simulink model "recycle1"  (R2024a)
settings: Solver=VariableStepAuto  StartTime=0.0  StopTime=100  MaxStep=0.1  RelTol=1e-3
libraries: simulink x20
(part 1 of 2)
settings Model: Creator=SEPTPFNK  LastModifiedBy=skoge
settings DataIOCC: SaveFormat=Array  SaveOutput=off  DSMLogging=off  ReturnWorkspaceOutputs=off  TimeSaveName=t
settings OptimizationCC: ReuseModelBlockBuffer=off
settings RTWCC: GPUComputeCapability=3.5

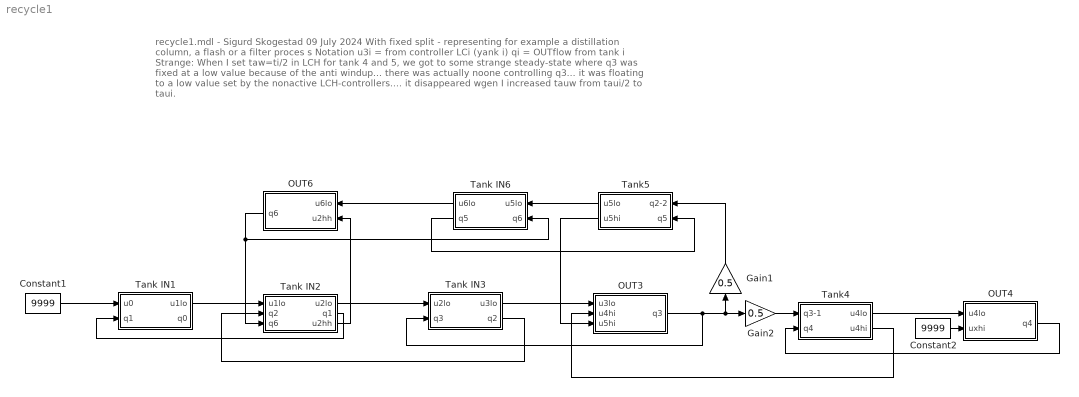
== system recycle1 ==
  note: recycle1.mdl - Sigurd Skogestad 09 July 2024
      | With fixed split - representing for example a distillation column, a flash or a filter proces s
      | Notation
      | u3i = from controller LCi (yank i)
      | qi = OUTflow from tank i
      |
      | Strange: When I set taw=ti/2 in LCH for tank 4 and 5, we got to some strange steady-state where q3 was fixed at a low value because of the anti windup... there was actually noone controlling q3... it was floating to a low value set by the nonactive LCH-controllers.... it disappeared wgen I increased tauw from taui/2 to taui.
  Constant1 : Constant  Value=9999
  Constant2 : Constant  Value=9999
  Gain1 : Gain  Gain=0.5  SaturateOnIntegerOverflow=on  OutDataTypeStr=Inherit: Same as input  ParamDataTypeStr=Inherit: Same as input
  Gain2 : Gain  Gain=0.5  SaturateOnIntegerOverflow=on  OutDataTypeStr=Inherit: Same as input  ParamDataTypeStr=Inherit: Same as input
  OUT3 : Subsystem
  OUT4 : Subsystem
  OUT6 : Subsystem
  Tank IN1 : Subsystem
  Tank IN2 : Subsystem
  Tank IN3 : Subsystem
  Tank IN6 : Subsystem
  Tank4 : Subsystem
  Tank5 : Subsystem
  wires:
  Tank IN1/1(u1lo) -> Tank IN2/1(u1lo)
  Tank IN2/2(q1) -> Tank IN1/2(q1)
  Constant1/1 -> Tank IN1/1(u0)
  Tank IN2/1(u2lo) -> Tank IN3/1(u2lo)
  Tank IN3/2(q2) -> Tank IN2/2(q2)
  Tank IN3/1(u3lo) -> OUT3/1(u3lo)
  OUT3/1(q3) -> Gain1/1, Gain2/1, Tank IN3/2(q3)
  Gain2/1 -> Tank4/1(q3-1)
  Tank4/1(u4lo) -> OUT4/1(u4lo)
  OUT4/1(q4) -> Tank4/2(q4)
  Constant2/1 -> OUT4/2(uxhi)
  Tank4/2(u4hi) -> OUT3/2(u4hi)
  Gain1/1 -> Tank5/1(q2-2)
  Tank5/2(u5hi) -> OUT3/3(u5hi)
  Tank5/1(u5lo) -> Tank IN6/1(u5lo)
  Tank IN6/2(q5) -> Tank5/2(q5)
  Tank IN6/1(u6lo) -> OUT6/1(u6lo)
  OUT6/1(q6) -> Tank IN2/3(q6), Tank IN6/2(q6)
  Tank IN2/3(u2hh) -> OUT6/2(u2hh)

== system recycle1/OUT3 ==
  note: This block represents an outflow valve and selector.
  note: Manual max-value; may represent bottleneck
  u3lo : Inport
  u4hi : Inport  Port=2
  u5hi : Inport  Port=3
  Constant2 : Constant  Value=9999
  Constant5 : Constant  Value=100
  Constant7 : Constant  Value=0
  SEL1 : MinMax  Inputs=4
  Saturation Dynamic : simulink/Discontinuities/Saturation Dynamic  OutMin=[]  OutMax=[]  OutDataTypeStr=Inherit: Same as second input  OutDataType=fixdt(1, 16)  OutScaling=2^-10  DoSatur=off
  Sum2 : Sum  Inputs=+++|
  ubq2 : Step  Time=120  After=-50  SampleTime=0
  ubq4 : Step  Time=100  After=10  SampleTime=0
  q3 : Outport
  wires:
  u3lo/1 -> SEL1/1
  SEL1/1 -> Saturation Dynamic/2
  Constant5/1 -> Saturation Dynamic/1
  Constant7/1 -> Saturation Dynamic/3
  Sum2/1 -> SEL1/2  "ubq4"
  Constant2/1 -> Sum2/1
  ubq2/1 -> Sum2/3
  ubq4/1 -> Sum2/2
  Saturation Dynamic/1 -> q3/1  "q3"
  u4hi/1 -> SEL1/3
  u5hi/1 -> SEL1/4

== system recycle1/OUT4 ==
  note: This block represents an outflow valve and selector.
  note: Manual max-value; may represent bottleneck
  u4lo : Inport
  uxhi : Inport  Port=2
  Constant2 : Constant  Value=9999
  Constant5 : Constant  Value=100
  Constant7 : Constant  Value=0
  SEL1 : MinMax  Inputs=3
  Saturation Dynamic : simulink/Discontinuities/Saturation Dynamic  OutMin=[]  OutMax=[]  OutDataTypeStr=Inherit: Same as second input  OutDataType=fixdt(1, 16)  OutScaling=2^-10  DoSatur=off
  Sum2 : Sum  Inputs=+++|
  ubq2 : Step  Time=40  After=-10  SampleTime=0
  ubq4 : Step  Time=10  After=0  SampleTime=0
  q4 : Outport
  wires:
  u4lo/1 -> SEL1/1
  SEL1/1 -> Saturation Dynamic/2
  Constant5/1 -> Saturation Dynamic/1
  Constant7/1 -> Saturation Dynamic/3
  Sum2/1 -> SEL1/2  "ubq5"
  Constant2/1 -> Sum2/1
  ubq2/1 -> Sum2/3
  ubq4/1 -> Sum2/2
  Saturation Dynamic/1 -> q4/1  "q4"
  uxhi/1 -> SEL1/3

== system recycle1/OUT6 ==
  note: This block represents an outflow valve and selector.
  note: Manual max-value; may represent bottleneck
  u6lo : Inport
  u2hh : Inport  Port=2
  Constant2 : Constant  Value=999
  Constant5 : Constant  Value=100
  Constant7 : Constant  Value=0
  SEL1 : MinMax  Inputs=3
  Saturation Dynamic : simulink/Discontinuities/Saturation Dynamic  OutMin=[]  OutMax=[]  OutDataTypeStr=Inherit: Same as second input  OutDataType=fixdt(1, 16)  OutScaling=2^-10  DoSatur=off
  Sum2 : Sum  Inputs=+++|
  ubq2 : Step  Time=40  After=-10  SampleTime=0
  ubq4 : Step  Time=10  After=0  SampleTime=0
  q6 : Outport
  wires:
  u6lo/1 -> SEL1/1
  SEL1/1 -> Saturation Dynamic/2
  Constant5/1 -> Saturation Dynamic/1
  Constant7/1 -> Saturation Dynamic/3
  Sum2/1 -> SEL1/2  "ubq5"
  Constant2/1 -> Sum2/1
  ubq2/1 -> Sum2/3
  ubq4/1 -> Sum2/2
  Saturation Dynamic/1 -> q6/1  "q7"
  u2hh/1 -> SEL1/3

== system recycle1/Tank IN1 ==
  note: This block represents a tank with bidirectional level control + inflow valve and selector.
  note: Manual max-value; may represent bottleneck
  u0 : Inport
  q1 : Inport  Port=2
  B2 : Integrator  InitialCondition=80  LimitOutput=on  UpperSaturationLimit=200  LowerSaturationLimit=-100
  Constant2 : Constant  Value=100
  Constant5 : Constant  Value=100
  Constant7 : Constant  Value=0
  LCH1 : Subsystem  mask(PID-controller){Kc=1, Ti=4, Tarw=4, r0=80, u0=80, yMin=0, yMax=100, uMin=0, uMax=100}
      mask prompts: Tarw "T_arw"; r0 "Setpoint:"; u0 "Initial output:"
      mask help: PID-controller
      mask Help:
      | <P> PID-controller with beta-factor, limiting, ARW etc </P>
      | 
      | Inputs: <P>
      |  <UL>
      |   1 = r (setpoint) <BR>
      |   2 = y (process value) <BR>
      |   3  = u0 (control signal offset) <BR>
      |  </UL>
      |  </P>
      | Outputs: <P>
      |  <UL>
      |    1 = u (control signal) <BR>
      |    2 = Proportional part  <BR>
      |    3 = Integral part  <BR>
      |    4 = Derivative part  <BR>
      |    5 = raw signal, without ARW  <BR>
      |  </UL>
      |  </P>
      mask Display:
      | disp(['PI' 10 10 10])
      | port_label('input',1,'y')
      | port_label('input',2,'uaw')
      | port_label('output',1,'u')
  LCL1 : Subsystem  mask(PID-controller){Kc=-1, Ti=4, Tarw=4, r0=10, u0=80, yMin=0, yMax=100, uMin=0, uMax=100}
      mask prompts: Tarw "T_arw"; r0 "Setpoint:"; u0 "Initial output:"
      mask help: PID-controller
      mask Help:
      | <P> PID-controller with beta-factor, limiting, ARW etc </P>
      | 
      | Inputs: <P>
      |  <UL>
      |   1 = r (setpoint) <BR>
      |   2 = y (process value) <BR>
      |   3  = u0 (control signal offset) <BR>
      |  </UL>
      |  </P>
      | Outputs: <P>
      |  <UL>
      |    1 = u (control signal) <BR>
      |    2 = Proportional part  <BR>
      |    3 = Integral part  <BR>
      |    4 = Derivative part  <BR>
      |    5 = raw signal, without ARW  <BR>
      |  </UL>
      |  </P>
      mask Display:
      | disp(['PI' 10 10 10])
      | port_label('input',1,'y')
      | port_label('input',2,'uaw')
      | port_label('output',1,'u')
  SEL1 : MinMax  Inputs=3
  Saturation Dynamic : simulink/Discontinuities/Saturation Dynamic  OutMin=[]  OutMax=[]  OutDataTypeStr=Inherit: Same as second input  OutDataType=fixdt(1, 16)  OutScaling=2^-10  DoSatur=off
  Sum1 : Sum  Inputs=|-+|
  Sum2 : Sum  Inputs=+++|
  ubq2 : Step  Time=120  After=-20  SampleTime=0
  ubq4 : Step  Time=40  After=-70  SampleTime=0
  u1lo : Outport
  q0 : Outport  Port=2
  wires:
  B2/1 -> LCL1/1(in_y), LCH1/1(in_y)  "x1"
  u0/1 -> SEL1/1
  SEL1/1 -> Saturation Dynamic/2
  Constant5/1 -> Saturation Dynamic/1
  LCH1/1(out_u) -> SEL1/3  "u1hi"
  Sum1/1 -> B2/1
  Constant7/1 -> Saturation Dynamic/3
  Saturation Dynamic/1 -> Sum1/2, q0/1, LCH1/2(in_yaw)  "q0"
  q1/1 -> LCL1/2(in_yaw), Sum1/1
  Sum2/1 -> SEL1/2  "ubq1"
  Constant2/1 -> Sum2/1
  ubq2/1 -> Sum2/3
  ubq4/1 -> Sum2/2
  LCL1/1(out_u) -> u1lo/1  "u1lo"

== system recycle1/Tank IN2 ==
  note: This block represents a tank with bidirectional level control + inflow valve and selector + t wo inflows (so one H and one HH setpoint)
  note: Manual max-value; may represent bottleneck
  u1lo : Inport
  q2 : Inport  Port=2
  q6 : Inport  Port=3
  B2 : Integrator  InitialCondition=80  LimitOutput=on  UpperSaturationLimit=200  LowerSaturationLimit=-100
  Constant2 : Constant  Value=9999
  Constant5 : Constant  Value=100
  Constant7 : Constant  Value=0
  LCH2 : Subsystem  mask(PID-controller){Kc=1, Ti=4, Tarw=4, r0=80, u0=80, yMin=0, yMax=100, uMin=0, uMax=100}
      mask prompts: Tarw "T_arw"; r0 "Setpoint:"; u0 "Initial output:"
      mask help: PID-controller
      mask Help:
      | <P> PID-controller with beta-factor, limiting, ARW etc </P>
      | 
      | Inputs: <P>
      |  <UL>
      |   1 = r (setpoint) <BR>
      |   2 = y (process value) <BR>
      |   3  = u0 (control signal offset) <BR>
      |  </UL>
      |  </P>
      | Outputs: <P>
      |  <UL>
      |    1 = u (control signal) <BR>
      |    2 = Proportional part  <BR>
      |    3 = Integral part  <BR>
      |    4 = Derivative part  <BR>
      |    5 = raw signal, without ARW  <BR>
      |  </UL>
      |  </P>
      mask Display:
      | disp(['PI' 10 10 10])
      | port_label('input',1,'y')
      | port_label('input',2,'uaw')
      | port_label('output',1,'u')
  LCHH2 : Subsystem  mask(PID-controller){Kc=1, Ti=4, Tarw=4, r0=90, u0=90, yMin=0, yMax=100, uMin=0, uMax=100}
      mask prompts: Tarw "T_arw"; r0 "Setpoint:"; u0 "Initial output:"
      mask help: PID-controller
      mask Help:
      | <P> PID-controller with beta-factor, limiting, ARW etc </P>
      | 
      | Inputs: <P>
      |  <UL>
      |   1 = r (setpoint) <BR>
      |   2 = y (process value) <BR>
      |   3  = u0 (control signal offset) <BR>
      |  </UL>
      |  </P>
      | Outputs: <P>
      |  <UL>
      |    1 = u (control signal) <BR>
      |    2 = Proportional part  <BR>
      |    3 = Integral part  <BR>
      |    4 = Derivative part  <BR>
      |    5 = raw signal, without ARW  <BR>
      |  </UL>
      |  </P>
      mask Display:
      | disp(['PI' 10 10 10])
      | port_label('input',1,'y')
      | port_label('input',2,'uaw')
      | port_label('output',1,'u')
  LCL2 : Subsystem  mask(PID-controller){Kc=-1, Ti=4, Tarw=4, r0=10, u0=80, yMin=0, yMax=100, uMin=0, uMax=100}
      mask prompts: Tarw "T_arw"; r0 "Setpoint:"; u0 "Initial output:"
      mask help: PID-controller
      mask Help:
      | <P> PID-controller with beta-factor, limiting, ARW etc </P>
      | 
      | Inputs: <P>
      |  <UL>
      |   1 = r (setpoint) <BR>
      |   2 = y (process value) <BR>
      |   3  = u0 (control signal offset) <BR>
      |  </UL>
      |  </P>
      | Outputs: <P>
      |  <UL>
      |    1 = u (control signal) <BR>
      |    2 = Proportional part  <BR>
      |    3 = Integral part  <BR>
      |    4 = Derivative part  <BR>
      |    5 = raw signal, without ARW  <BR>
      |  </UL>
      |  </P>
      mask Display:
      | disp(['PI' 10 10 10])
      | port_label('input',1,'y')
      | port_label('input',2,'uaw')
      | port_label('output',1,'u')
  SEL1 : MinMax  Inputs=3
  Saturation Dynamic : simulink/Discontinuities/Saturation Dynamic  OutMin=[]  OutMax=[]  OutDataTypeStr=Inherit: Same as second input  OutDataType=fixdt(1, 16)  OutScaling=2^-10  DoSatur=off
  Sum1 : Sum  Inputs=|-++|
  Sum2 : Sum  Inputs=+++|
  ubq2 : Step  Time=120  After=-20  SampleTime=0
  ubq4 : Step  Time=102  After=20  SampleTime=0
  u2lo : Outport
  q1 : Outport  Port=2
  u2hh : Outport  Port=3
  wires:
  B2/1 -> LCHH2/1(in_y), LCL2/1(in_y), LCH2/1(in_y)  "x2"
  u1lo/1 -> SEL1/1
  SEL1/1 -> Saturation Dynamic/2
  Constant5/1 -> Saturation Dynamic/1
  LCH2/1(out_u) -> SEL1/3  "u2hi"
  Sum1/1 -> B2/1
  Constant7/1 -> Saturation Dynamic/3
  Saturation Dynamic/1 -> LCH2/2(in_yaw), Sum1/2, q1/1  "q1"
  q2/1 -> LCL2/2(in_yaw), Sum1/1
  Sum2/1 -> SEL1/2  "ubq2"
  Constant2/1 -> Sum2/1
  ubq2/1 -> Sum2/3
  ubq4/1 -> Sum2/2
  LCL2/1(out_u) -> u2lo/1  "u2lo"
  LCHH2/1(out_u) -> u2hh/1  "u2hh"
  q6/1 -> LCHH2/2(in_yaw), Sum1/3

== system recycle1/Tank IN3 ==
  note: This block represents a tank with bidirectional level control + inflow valve and selector.
  note: Manual max-value; may represent bottleneck
  u2lo : Inport
  q3 : Inport  Port=2
  B3 : Integrator  InitialCondition=80  LimitOutput=on  UpperSaturationLimit=200  LowerSaturationLimit=-100
  Constant2 : Constant  Value=9999
  Constant5 : Constant  Value=100
  Constant7 : Constant  Value=0
  LCH3 : Subsystem  mask(PID-controller){Kc=1, Ti=4, Tarw=4, r0=80, u0=80, yMin=0, yMax=100, uMin=0, uMax=100}
      mask prompts: Tarw "T_arw"; r0 "Setpoint:"; u0 "Initial output:"
      mask help: PID-controller
      mask Help:
      | <P> PID-controller with beta-factor, limiting, ARW etc </P>
      | 
      | Inputs: <P>
      |  <UL>
      |   1 = r (setpoint) <BR>
      |   2 = y (process value) <BR>
      |   3  = u0 (control signal offset) <BR>
      |  </UL>
      |  </P>
      | Outputs: <P>
      |  <UL>
      |    1 = u (control signal) <BR>
      |    2 = Proportional part  <BR>
      |    3 = Integral part  <BR>
      |    4 = Derivative part  <BR>
      |    5 = raw signal, without ARW  <BR>
      |  </UL>
      |  </P>
      mask Display:
      | disp(['PI' 10 10 10])
      | port_label('input',1,'y')
      | port_label('input',2,'uaw')
      | port_label('output',1,'u')
  LCL3 : Subsystem  mask(PID-controller){Kc=-1, Ti=4, Tarw=4, r0=10, u0=80, yMin=0, yMax=100, uMin=0, uMax=100}
      mask prompts: Tarw "T_arw"; r0 "Setpoint:"; u0 "Initial output:"
      mask help: PID-controller
      mask Help:
      | <P> PID-controller with beta-factor, limiting, ARW etc </P>
      | 
      | Inputs: <P>
      |  <UL>
      |   1 = r (setpoint) <BR>
      |   2 = y (process value) <BR>
      |   3  = u0 (control signal offset) <BR>
      |  </UL>
      |  </P>
      | Outputs: <P>
      |  <UL>
      |    1 = u (control signal) <BR>
      |    2 = Proportional part  <BR>
      |    3 = Integral part  <BR>
      |    4 = Derivative part  <BR>
      |    5 = raw signal, without ARW  <BR>
      |  </UL>
      |  </P>
      mask Display:
      | disp(['PI' 10 10 10])
      | port_label('input',1,'y')
      | port_label('input',2,'uaw')
      | port_label('output',1,'u')
  SEL1 : MinMax  Inputs=3
  Saturation Dynamic : simulink/Discontinuities/Saturation Dynamic  OutMin=[]  OutMax=[]  OutDataTypeStr=Inherit: Same as second input  OutDataType=fixdt(1, 16)  OutScaling=2^-10  DoSatur=off
  Sum1 : Sum  Inputs=|-+|
  Sum2 : Sum  Inputs=+++|
  ubq2 : Step  Time=20  After=-60  SampleTime=0
  ubq4 : Step  Time=10  After=20  SampleTime=0
  u3lo : Outport
  q2 : Outport  Port=2
  wires:
  B3/1 -> LCH3/1(in_y), LCL3/1(in_y)  "x3"
  u2lo/1 -> SEL1/1
  SEL1/1 -> Saturation Dynamic/2
  Constant5/1 -> Saturation Dynamic/1
  LCH3/1(out_u) -> SEL1/3  "u3hi"
  Sum1/1 -> B3/1
  Constant7/1 -> Saturation Dynamic/3
  Saturation Dynamic/1 -> LCH3/2(in_yaw), Sum1/2, q2/1  "q2"
  q3/1 -> LCL3/2(in_yaw), Sum1/1
  Sum2/1 -> SEL1/2  "ubq3"
  Constant2/1 -> Sum2/1
  ubq2/1 -> Sum2/3
  ubq4/1 -> Sum2/2
  LCL3/1(out_u) -> u3lo/1  "u3lo"

== system recycle1/Tank IN6 ==
  note: This block represents a tank with bidirectional level control + inflow valve and selector.
  note: Manual max-value; may represent bottleneck
  u5lo : Inport
  q6 : Inport  Port=2
  B6 : Integrator  InitialCondition=10  LimitOutput=on  UpperSaturationLimit=200  LowerSaturationLimit=-100
  Constant2 : Constant  Value=100
  Constant5 : Constant  Value=100
  Constant7 : Constant  Value=0
  LCH6 : Subsystem  mask(PID-controller){Kc=1, Ti=4, Tarw=4, r0=80, u0=80, yMin=0, yMax=100, uMin=0, uMax=100}
      mask prompts: Tarw "T_arw"; r0 "Setpoint:"; u0 "Initial output:"
      mask help: PID-controller
      mask Help:
      | <P> PID-controller with beta-factor, limiting, ARW etc </P>
      | 
      | Inputs: <P>
      |  <UL>
      |   1 = r (setpoint) <BR>
      |   2 = y (process value) <BR>
      |   3  = u0 (control signal offset) <BR>
      |  </UL>
      |  </P>
      | Outputs: <P>
      |  <UL>
      |    1 = u (control signal) <BR>
      |    2 = Proportional part  <BR>
      |    3 = Integral part  <BR>
      |    4 = Derivative part  <BR>
      |    5 = raw signal, without ARW  <BR>
      |  </UL>
      |  </P>
      mask Display:
      | disp(['PI' 10 10 10])
      | port_label('input',1,'y')
      | port_label('input',2,'uaw')
      | port_label('output',1,'u')
  LCL6 : Subsystem  mask(PID-controller){Kc=-1, Ti=4, Tarw=4, r0=10, u0=80, yMin=0, yMax=100, uMin=0, uMax=100}
      mask prompts: Tarw "T_arw"; r0 "Setpoint:"; u0 "Initial output:"
      mask help: PID-controller
      mask Help:
      | <P> PID-controller with beta-factor, limiting, ARW etc </P>
      | 
      | Inputs: <P>
      |  <UL>
      |   1 = r (setpoint) <BR>
      |   2 = y (process value) <BR>
      |   3  = u0 (control signal offset) <BR>
      |  </UL>
      |  </P>
      | Outputs: <P>
      |  <UL>
      |    1 = u (control signal) <BR>
      |    2 = Proportional part  <BR>
      |    3 = Integral part  <BR>
      |    4 = Derivative part  <BR>
      |    5 = raw signal, without ARW  <BR>
      |  </UL>
      |  </P>
      mask Display:
      | disp(['PI' 10 10 10])
      | port_label('input',1,'y')
      | port_label('input',2,'uaw')
      | port_label('output',1,'u')
  SEL1 : MinMax  Inputs=3
  Saturation Dynamic : simulink/Discontinuities/Saturation Dynamic  OutMin=[]  OutMax=[]  OutDataTypeStr=Inherit: Same as second input  OutDataType=fixdt(1, 16)  OutScaling=2^-10  DoSatur=off
  Sum1 : Sum  Inputs=|-+|
  Sum2 : Sum  Inputs=+++|
  ubq2 : Step  Time=200  After=-60  SampleTime=0
  ubq4 : Step  Time=60  After=-90  SampleTime=0
  u6lo : Outport
  q5 : Outport  Port=2
  wires:
  B6/1 -> LCH6/1(in_y), LCL6/1(in_y)  "x6"
  u5lo/1 -> SEL1/1
  SEL1/1 -> Saturation Dynamic/2
  Constant5/1 -> Saturation Dynamic/1
  LCH6/1(out_u) -> SEL1/3  "u6hi"
  Sum1/1 -> B6/1
  Constant7/1 -> Saturation Dynamic/3
  Saturation Dynamic/1 -> LCH6/2(in_yaw), Sum1/2, q5/1  "q5"
  q6/1 -> LCL6/2(in_yaw), Sum1/1
  Sum2/1 -> SEL1/2  "ubq6"
  Constant2/1 -> Sum2/1
  ubq2/1 -> Sum2/3
  ubq4/1 -> Sum2/2
  LCL6/1(out_u) -> u6lo/1  "u6lo"

== system recycle1/Tank4 ==
  note: This block represents a tank with bidirectional level control .
  q3-1 : Inport
  q4 : Inport  Port=2
  B4 : Integrator  InitialCondition=10  LimitOutput=on  UpperSaturationLimit=200  LowerSaturationLimit=-100
  LCH4 : Subsystem  mask(PID-controller){Kc=1, Ti=4, Tarw=4, r0=80, u0=80, yMin=0, yMax=100, uMin=0, uMax=100}
      mask prompts: Tarw "T_arw"; r0 "Setpoint:"; u0 "Initial output:"
      mask help: PID-controller
      mask Help:
      | <P> PID-controller with beta-factor, limiting, ARW etc </P>
      | 
      | Inputs: <P>
      |  <UL>
      |   1 = r (setpoint) <BR>
      |   2 = y (process value) <BR>
      |   3  = u0 (control signal offset) <BR>
      |  </UL>
      |  </P>
      | Outputs: <P>
      |  <UL>
      |    1 = u (control signal) <BR>
      |    2 = Proportional part  <BR>
      |    3 = Integral part  <BR>
      |    4 = Derivative part  <BR>
      |    5 = raw signal, without ARW  <BR>
      |  </UL>
      |  </P>
      mask Display:
      | disp(['PI' 10 10 10])
      | port_label('input',1,'y')
      | port_label('input',2,'uaw')
      | port_label('output',1,'u')
  LCL4 : Subsystem  mask(PID-controller){Kc=-1, Ti=4, Tarw=4, r0=10, u0=80, yMin=0, yMax=100, uMin=0, uMax=100}
      mask prompts: Tarw "T_arw"; r0 "Setpoint:"; u0 "Initial output:"
      mask help: PID-controller
      mask Help:
      | <P> PID-controller with beta-factor, limiting, ARW etc </P>
      | 
      | Inputs: <P>
      |  <UL>
      |   1 = r (setpoint) <BR>
      |   2 = y (process value) <BR>
      |   3  = u0 (control signal offset) <BR>
      |  </UL>
      |  </P>
      | Outputs: <P>
      |  <UL>
      |    1 = u (control signal) <BR>
      |    2 = Proportional part  <BR>
      |    3 = Integral part  <BR>
      |    4 = Derivative part  <BR>
      |    5 = raw signal, without ARW  <BR>
      |  </UL>
      |  </P>
      mask Display:
      | disp(['PI' 10 10 10])
      | port_label('input',1,'y')
      | port_label('input',2,'uaw')
      | port_label('output',1,'u')
  Sum1 : Sum  Inputs=|-+|
  u4lo : Outport
  u4hi : Outport  Port=2
  wires:
  B4/1 -> LCH4/1(in_y), LCL4/1(in_y)  "x4"
  LCH4/1(out_u) -> u4hi/1  "u4hi"
  Sum1/1 -> B4/1
  q4/1 -> LCL4/2(in_yaw), Sum1/1
  LCL4/1(out_u) -> u4lo/1  "u4lo"
  q3-1/1 -> LCH4/2(in_yaw), Sum1/2

== system recycle1/Tank5 ==
  note: This block represents a tank with bidirectional level control .
  q2-2 : Inport
  q5 : Inport  Port=2
  B5 : Integrator  InitialCondition=10  LimitOutput=on  UpperSaturationLimit=200  LowerSaturationLimit=-100
  LCH5 : Subsystem  mask(PID-controller){Kc=1, Ti=4, Tarw=4, r0=80, u0=80, yMin=0, yMax=100, uMin=0, uMax=100}
      mask prompts: Tarw "T_arw"; r0 "Setpoint:"; u0 "Initial output:"
      mask help: PID-controller
      mask Help:
      | <P> PID-controller with beta-factor, limiting, ARW etc </P>
      | 
      | Inputs: <P>
      |  <UL>
      |   1 = r (setpoint) <BR>
      |   2 = y (process value) <BR>
      |   3  = u0 (control signal offset) <BR>
      |  </UL>
      |  </P>
      | Outputs: <P>
      |  <UL>
      |    1 = u (control signal) <BR>
      |    2 = Proportional part  <BR>
      |    3 = Integral part  <BR>
      |    4 = Derivative part  <BR>
      |    5 = raw signal, without ARW  <BR>
      |  </UL>
      |  </P>
      mask Display:
      | disp(['PI' 10 10 10])
      | port_label('input',1,'y')
      | port_label('input',2,'uaw')
      | port_label('output',1,'u')
  LCL5 : Subsystem  mask(PID-controller){Kc=-1, Ti=4, Tarw=4, r0=10, u0=80, yMin=0, yMax=100, uMin=0, uMax=100}
      mask prompts: Tarw "T_arw"; r0 "Setpoint:"; u0 "Initial output:"
      mask help: PID-controller
      mask Help:
      | <P> PID-controller with beta-factor, limiting, ARW etc </P>
      | 
      | Inputs: <P>
      |  <UL>
      |   1 = r (setpoint) <BR>
      |   2 = y (process value) <BR>
      |   3  = u0 (control signal offset) <BR>
      |  </UL>
      |  </P>
      | Outputs: <P>
      |  <UL>
      |    1 = u (control signal) <BR>
      |    2 = Proportional part  <BR>
      |    3 = Integral part  <BR>
      |    4 = Derivative part  <BR>
      |    5 = raw signal, without ARW  <BR>
      |  </UL>
      |  </P>
      mask Display:
      | disp(['PI' 10 10 10])
      | port_label('input',1,'y')
      | port_label('input',2,'uaw')
      | port_label('output',1,'u')
  Sum1 : Sum  Inputs=|-+|
  u5lo : Outport
  u5hi : Outport  Port=2
  wires:
  B5/1 -> LCH5/1(in_y), LCL5/1(in_y)  "x5"
  LCH5/1(out_u) -> u5hi/1  "u5hi"
  Sum1/1 -> B5/1
  q5/1 -> LCL5/2(in_yaw), Sum1/1
  LCL5/1(out_u) -> u5lo/1  "u5lo"
  q2-2/1 -> LCH5/2(in_yaw), Sum1/2

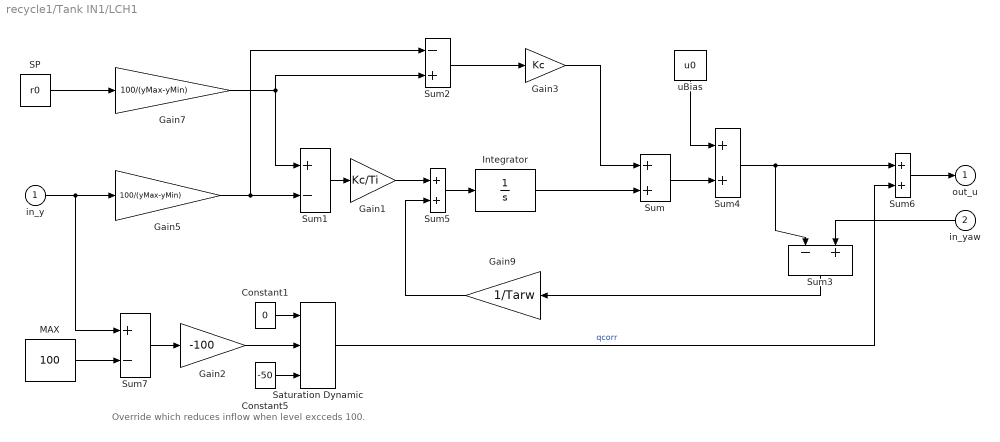
== system recycle1/Tank IN1/LCH1 ==
  note: Override which reduces inflow when level excceds 100.
  in_y : Inport
  in_yaw : Inport  Port=2
  Constant1 : Constant  Value=0
  Constant5 : Constant  Value=-50
  Gain1 : Gain  Gain=Kc/Ti  SaturateOnIntegerOverflow=on  OutDataTypeStr=Inherit: Same as input  ParamDataTypeStr=Inherit: Same as input
  Gain2 : Gain  Gain=-100  SaturateOnIntegerOverflow=on  OutDataTypeStr=Inherit: Same as input  ParamDataTypeStr=Inherit: Same as input
  Gain3 : Gain  Gain=Kc  SaturateOnIntegerOverflow=on  OutDataTypeStr=Inherit: Same as input  ParamDataTypeStr=Inherit: Same as input
  Gain5 : Gain  Gain=100/(yMax-yMin)  SaturateOnIntegerOverflow=on  OutDataTypeStr=Inherit: Same as input  ParamDataTypeStr=Inherit: Same as input
  Gain7 : Gain  Gain=100/(yMax-yMin)  SaturateOnIntegerOverflow=on  OutDataTypeStr=Inherit: Same as input  ParamDataTypeStr=Inherit: Same as input
  Gain9 : Gain  Gain=1/Tarw  SaturateOnIntegerOverflow=on  OutDataTypeStr=Inherit: Same as input  ParamDataTypeStr=Inherit: Same as input
  Integrator : Integrator
  MAX : Constant  Value=100
  SP : Constant  Value=r0
  Saturation Dynamic : simulink/Discontinuities/Saturation Dynamic  OutMin=[]  OutMax=[]  OutDataTypeStr=Inherit: Same as second input  OutDataType=fixdt(1, 16)  OutScaling=2^-10  DoSatur=off
  Sum{,4..6} (4 alike) : Sum  InputSameDT=on  SaturateOnIntegerOverflow=on  OutDataTypeStr=Inherit: Same as first input
  Sum1 : Sum  Inputs=+-  InputSameDT=on  SaturateOnIntegerOverflow=on  OutDataTypeStr=Inherit: Same as first input
  Sum2 : Sum  Inputs=-+  InputSameDT=on  SaturateOnIntegerOverflow=on  OutDataTypeStr=Inherit: Same as first input
  Sum3 : Sum  Inputs=-+  InputSameDT=on  SaturateOnIntegerOverflow=on  OutDataTypeStr=Inherit: Same as first input
  Sum7 : Sum  Inputs=+-  InputSameDT=on  SaturateOnIntegerOverflow=on  OutDataTypeStr=Inherit: Same as first input
  uBias : Constant  Value=u0
  out_u : Outport  VectorParamsAs1DForOutWhenUnconnected=off
  wires:
  Gain3/1 -> Sum/1
  Sum5/1 -> Integrator/1
  Gain9/1 -> Sum5/2
  Gain1/1 -> Sum5/1
  Sum3/1 -> Gain9/1
  Sum/1 -> Sum4/2
  Sum4/1 -> Sum6/1, Sum3/1
  Gain5/1 -> Sum2/1, Sum1/2
  Sum2/1 -> Gain3/1
  Gain7/1 -> Sum2/2, Sum1/1
  Sum1/1 -> Gain1/1
  in_y/1 -> Sum7/1, Gain5/1
  SP/1 -> Gain7/1
  Integrator/1 -> Sum/2
  uBias/1 -> Sum4/1
  in_yaw/1 -> Sum3/2
  Gain2/1 -> Saturation Dynamic/2
  Constant1/1 -> Saturation Dynamic/1
  Constant5/1 -> Saturation Dynamic/3
  Sum6/1 -> out_u/1
  Saturation Dynamic/1 -> Sum6/2  "qcorr"
  Sum7/1 -> Gain2/1
  MAX/1 -> Sum7/2

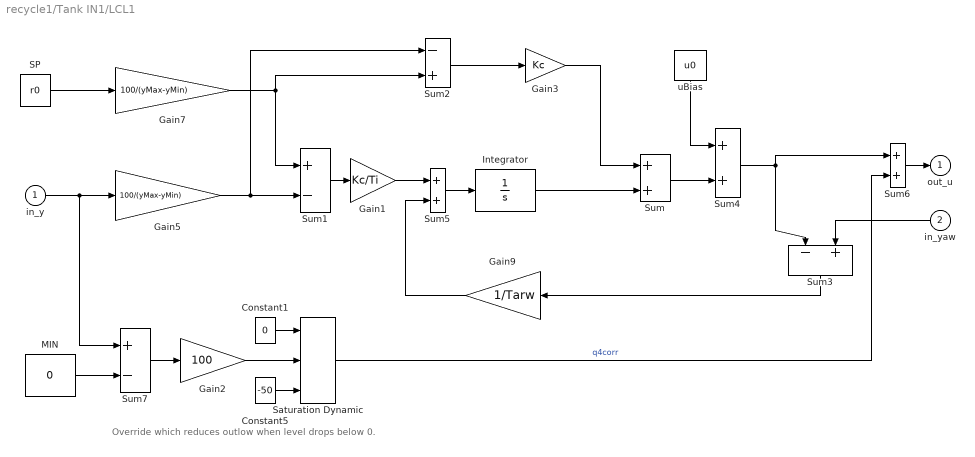
== system recycle1/Tank IN1/LCL1 ==
  note: Override which reduces outlow when level drops below 0.
  in_y : Inport
  in_yaw : Inport  Port=2
  Constant1 : Constant  Value=0
  Constant5 : Constant  Value=-50
  Gain1 : Gain  Gain=Kc/Ti  SaturateOnIntegerOverflow=on  OutDataTypeStr=Inherit: Same as input  ParamDataTypeStr=Inherit: Same as input
  Gain2 : Gain  Gain=100  SaturateOnIntegerOverflow=on  OutDataTypeStr=Inherit: Same as input  ParamDataTypeStr=Inherit: Same as input
  Gain3 : Gain  Gain=Kc  SaturateOnIntegerOverflow=on  OutDataTypeStr=Inherit: Same as input  ParamDataTypeStr=Inherit: Same as input
  Gain5 : Gain  Gain=100/(yMax-yMin)  SaturateOnIntegerOverflow=on  OutDataTypeStr=Inherit: Same as input  ParamDataTypeStr=Inherit: Same as input
  Gain7 : Gain  Gain=100/(yMax-yMin)  SaturateOnIntegerOverflow=on  OutDataTypeStr=Inherit: Same as input  ParamDataTypeStr=Inherit: Same as input
  Gain9 : Gain  Gain=1/Tarw  SaturateOnIntegerOverflow=on  OutDataTypeStr=Inherit: Same as input  ParamDataTypeStr=Inherit: Same as input
  Integrator : Integrator
  MIN : Constant  Value=0
  SP : Constant  Value=r0
  Saturation Dynamic : simulink/Discontinuities/Saturation Dynamic  OutMin=[]  OutMax=[]  OutDataTypeStr=Inherit: Same as second input  OutDataType=fixdt(1, 16)  OutScaling=2^-10  DoSatur=off
  Sum{,4..6} (4 alike) : Sum  InputSameDT=on  SaturateOnIntegerOverflow=on  OutDataTypeStr=Inherit: Same as first input
  Sum1 : Sum  Inputs=+-  InputSameDT=on  SaturateOnIntegerOverflow=on  OutDataTypeStr=Inherit: Same as first input
  Sum2 : Sum  Inputs=-+  InputSameDT=on  SaturateOnIntegerOverflow=on  OutDataTypeStr=Inherit: Same as first input
  Sum3 : Sum  Inputs=-+  InputSameDT=on  SaturateOnIntegerOverflow=on  OutDataTypeStr=Inherit: Same as first input
  Sum7 : Sum  Inputs=+-  InputSameDT=on  SaturateOnIntegerOverflow=on  OutDataTypeStr=Inherit: Same as first input
  uBias : Constant  Value=u0
  out_u : Outport  VectorParamsAs1DForOutWhenUnconnected=off
  wires:
  Gain3/1 -> Sum/1
  Sum5/1 -> Integrator/1
  Gain9/1 -> Sum5/2
  Gain1/1 -> Sum5/1
  Sum3/1 -> Gain9/1
  Sum/1 -> Sum4/2
  Gain5/1 -> Sum2/1, Sum1/2
  Sum2/1 -> Gain3/1
  Gain7/1 -> Sum2/2, Sum1/1
  Sum1/1 -> Gain1/1
  in_y/1 -> Sum7/1, Gain5/1
  SP/1 -> Gain7/1
  Integrator/1 -> Sum/2
  uBias/1 -> Sum4/1
  in_yaw/1 -> Sum3/2
  Constant5/1 -> Saturation Dynamic/3
  Saturation Dynamic/1 -> Sum6/2  "q4corr"
  MIN/1 -> Sum7/2
  Gain2/1 -> Saturation Dynamic/2
  Sum7/1 -> Gain2/1
  Constant1/1 -> Saturation Dynamic/1
  Sum4/1 -> Sum3/1, Sum6/1
  Sum6/1 -> out_u/1

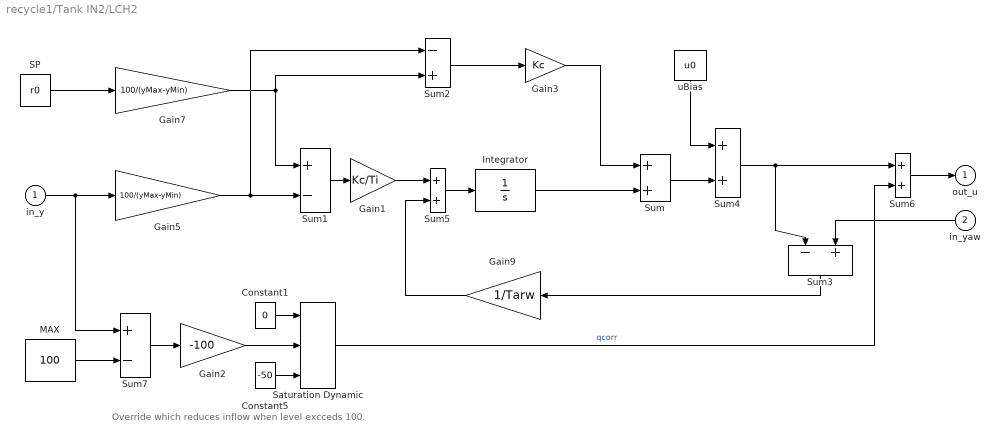
== system recycle1/Tank IN2/LCH2 ==
  note: Override which reduces inflow when level excceds 100.
  in_y : Inport
  in_yaw : Inport  Port=2
  Constant1 : Constant  Value=0
  Constant5 : Constant  Value=-50
  Gain1 : Gain  Gain=Kc/Ti  SaturateOnIntegerOverflow=on  OutDataTypeStr=Inherit: Same as input  ParamDataTypeStr=Inherit: Same as input
  Gain2 : Gain  Gain=-100  SaturateOnIntegerOverflow=on  OutDataTypeStr=Inherit: Same as input  ParamDataTypeStr=Inherit: Same as input
  Gain3 : Gain  Gain=Kc  SaturateOnIntegerOverflow=on  OutDataTypeStr=Inherit: Same as input  ParamDataTypeStr=Inherit: Same as input
  Gain5 : Gain  Gain=100/(yMax-yMin)  SaturateOnIntegerOverflow=on  OutDataTypeStr=Inherit: Same as input  ParamDataTypeStr=Inherit: Same as input
  Gain7 : Gain  Gain=100/(yMax-yMin)  SaturateOnIntegerOverflow=on  OutDataTypeStr=Inherit: Same as input  ParamDataTypeStr=Inherit: Same as input
  Gain9 : Gain  Gain=1/Tarw  SaturateOnIntegerOverflow=on  OutDataTypeStr=Inherit: Same as input  ParamDataTypeStr=Inherit: Same as input
  Integrator : Integrator
  MAX : Constant  Value=100
  SP : Constant  Value=r0
  Saturation Dynamic : simulink/Discontinuities/Saturation Dynamic  OutMin=[]  OutMax=[]  OutDataTypeStr=Inherit: Same as second input  OutDataType=fixdt(1, 16)  OutScaling=2^-10  DoSatur=off
  Sum{,4..6} (4 alike) : Sum  InputSameDT=on  SaturateOnIntegerOverflow=on  OutDataTypeStr=Inherit: Same as first input
  Sum1 : Sum  Inputs=+-  InputSameDT=on  SaturateOnIntegerOverflow=on  OutDataTypeStr=Inherit: Same as first input
  Sum2 : Sum  Inputs=-+  InputSameDT=on  SaturateOnIntegerOverflow=on  OutDataTypeStr=Inherit: Same as first input
  Sum3 : Sum  Inputs=-+  InputSameDT=on  SaturateOnIntegerOverflow=on  OutDataTypeStr=Inherit: Same as first input
  Sum7 : Sum  Inputs=+-  InputSameDT=on  SaturateOnIntegerOverflow=on  OutDataTypeStr=Inherit: Same as first input
  uBias : Constant  Value=u0
  out_u : Outport  VectorParamsAs1DForOutWhenUnconnected=off
  wires:
  Gain3/1 -> Sum/1
  Sum5/1 -> Integrator/1
  Gain9/1 -> Sum5/2
  Gain1/1 -> Sum5/1
  Sum3/1 -> Gain9/1
  Sum/1 -> Sum4/2
  Sum4/1 -> Sum6/1, Sum3/1
  Gain5/1 -> Sum2/1, Sum1/2
  Sum2/1 -> Gain3/1
  Gain7/1 -> Sum2/2, Sum1/1
  Sum1/1 -> Gain1/1
  in_y/1 -> Sum7/1, Gain5/1
  SP/1 -> Gain7/1
  Integrator/1 -> Sum/2
  uBias/1 -> Sum4/1
  in_yaw/1 -> Sum3/2
  Gain2/1 -> Saturation Dynamic/2
  Constant1/1 -> Saturation Dynamic/1
  Constant5/1 -> Saturation Dynamic/3
  Sum6/1 -> out_u/1
  Saturation Dynamic/1 -> Sum6/2  "qcorr"
  Sum7/1 -> Gain2/1
  MAX/1 -> Sum7/2

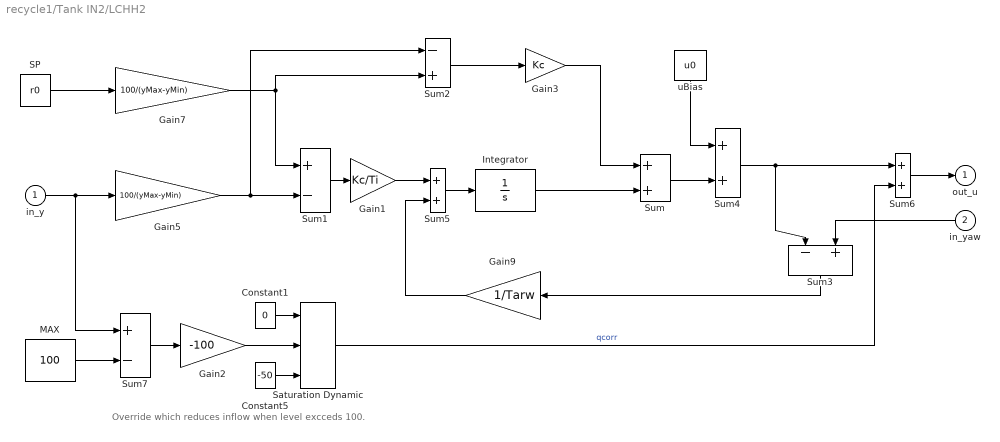
== system recycle1/Tank IN2/LCHH2 ==
  note: Override which reduces inflow when level excceds 100.
  in_y : Inport
  in_yaw : Inport  Port=2
  Constant1 : Constant  Value=0
  Constant5 : Constant  Value=-50
  Gain1 : Gain  Gain=Kc/Ti  SaturateOnIntegerOverflow=on  OutDataTypeStr=Inherit: Same as input  ParamDataTypeStr=Inherit: Same as input
  Gain2 : Gain  Gain=-100  SaturateOnIntegerOverflow=on  OutDataTypeStr=Inherit: Same as input  ParamDataTypeStr=Inherit: Same as input
  Gain3 : Gain  Gain=Kc  SaturateOnIntegerOverflow=on  OutDataTypeStr=Inherit: Same as input  ParamDataTypeStr=Inherit: Same as input
  Gain5 : Gain  Gain=100/(yMax-yMin)  SaturateOnIntegerOverflow=on  OutDataTypeStr=Inherit: Same as input  ParamDataTypeStr=Inherit: Same as input
  Gain7 : Gain  Gain=100/(yMax-yMin)  SaturateOnIntegerOverflow=on  OutDataTypeStr=Inherit: Same as input  ParamDataTypeStr=Inherit: Same as input
  Gain9 : Gain  Gain=1/Tarw  SaturateOnIntegerOverflow=on  OutDataTypeStr=Inherit: Same as input  ParamDataTypeStr=Inherit: Same as input
  Integrator : Integrator
  MAX : Constant  Value=100
  SP : Constant  Value=r0
  Saturation Dynamic : simulink/Discontinuities/Saturation Dynamic  OutMin=[]  OutMax=[]  OutDataTypeStr=Inherit: Same as second input  OutDataType=fixdt(1, 16)  OutScaling=2^-10  DoSatur=off
  Sum{,4..6} (4 alike) : Sum  InputSameDT=on  SaturateOnIntegerOverflow=on  OutDataTypeStr=Inherit: Same as first input
  Sum1 : Sum  Inputs=+-  InputSameDT=on  SaturateOnIntegerOverflow=on  OutDataTypeStr=Inherit: Same as first input
  Sum2 : Sum  Inputs=-+  InputSameDT=on  SaturateOnIntegerOverflow=on  OutDataTypeStr=Inherit: Same as first input
  Sum3 : Sum  Inputs=-+  InputSameDT=on  SaturateOnIntegerOverflow=on  OutDataTypeStr=Inherit: Same as first input
  Sum7 : Sum  Inputs=+-  InputSameDT=on  SaturateOnIntegerOverflow=on  OutDataTypeStr=Inherit: Same as first input
  uBias : Constant  Value=u0
  out_u : Outport  VectorParamsAs1DForOutWhenUnconnected=off
  wires:
  Gain3/1 -> Sum/1
  Sum5/1 -> Integrator/1
  Gain9/1 -> Sum5/2
  Gain1/1 -> Sum5/1
  Sum3/1 -> Gain9/1
  Sum/1 -> Sum4/2
  Sum4/1 -> Sum6/1, Sum3/1
  Gain5/1 -> Sum2/1, Sum1/2
  Sum2/1 -> Gain3/1
  Gain7/1 -> Sum2/2, Sum1/1
  Sum1/1 -> Gain1/1
  in_y/1 -> Sum7/1, Gain5/1
  SP/1 -> Gain7/1
  Integrator/1 -> Sum/2
  uBias/1 -> Sum4/1
  in_yaw/1 -> Sum3/2
  Gain2/1 -> Saturation Dynamic/2
  Constant1/1 -> Saturation Dynamic/1
  Constant5/1 -> Saturation Dynamic/3
  Sum6/1 -> out_u/1
  Saturation Dynamic/1 -> Sum6/2  "qcorr"
  Sum7/1 -> Gain2/1
  MAX/1 -> Sum7/2

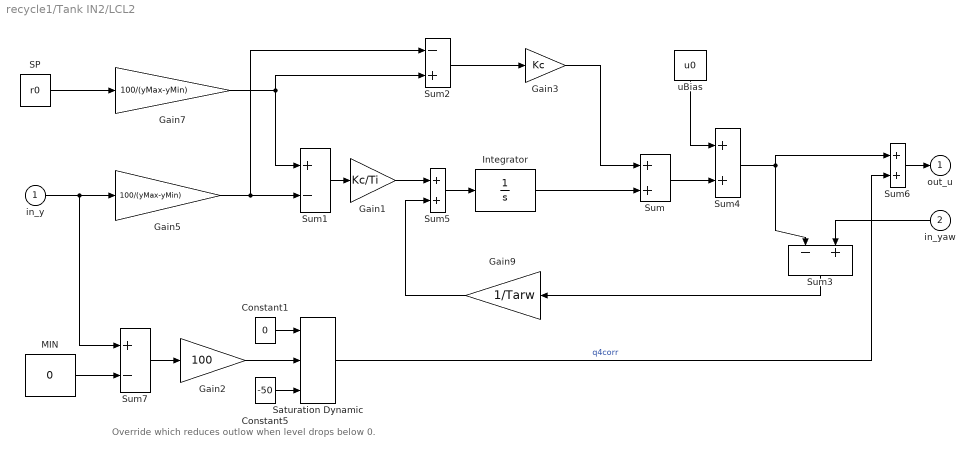
== system recycle1/Tank IN2/LCL2 ==
  note: Override which reduces outlow when level drops below 0.
  in_y : Inport
  in_yaw : Inport  Port=2
  Constant1 : Constant  Value=0
  Constant5 : Constant  Value=-50
  Gain1 : Gain  Gain=Kc/Ti  SaturateOnIntegerOverflow=on  OutDataTypeStr=Inherit: Same as input  ParamDataTypeStr=Inherit: Same as input
  Gain2 : Gain  Gain=100  SaturateOnIntegerOverflow=on  OutDataTypeStr=Inherit: Same as input  ParamDataTypeStr=Inherit: Same as input
  Gain3 : Gain  Gain=Kc  SaturateOnIntegerOverflow=on  OutDataTypeStr=Inherit: Same as input  ParamDataTypeStr=Inherit: Same as input
  Gain5 : Gain  Gain=100/(yMax-yMin)  SaturateOnIntegerOverflow=on  OutDataTypeStr=Inherit: Same as input  ParamDataTypeStr=Inherit: Same as input
  Gain7 : Gain  Gain=100/(yMax-yMin)  SaturateOnIntegerOverflow=on  OutDataTypeStr=Inherit: Same as input  ParamDataTypeStr=Inherit: Same as input
  Gain9 : Gain  Gain=1/Tarw  SaturateOnIntegerOverflow=on  OutDataTypeStr=Inherit: Same as input  ParamDataTypeStr=Inherit: Same as input
  Integrator : Integrator
  MIN : Constant  Value=0
  SP : Constant  Value=r0
  Saturation Dynamic : simulink/Discontinuities/Saturation Dynamic  OutMin=[]  OutMax=[]  OutDataTypeStr=Inherit: Same as second input  OutDataType=fixdt(1, 16)  OutScaling=2^-10  DoSatur=off
  Sum{,4..6} (4 alike) : Sum  InputSameDT=on  SaturateOnIntegerOverflow=on  OutDataTypeStr=Inherit: Same as first input
  Sum1 : Sum  Inputs=+-  InputSameDT=on  SaturateOnIntegerOverflow=on  OutDataTypeStr=Inherit: Same as first input
  Sum2 : Sum  Inputs=-+  InputSameDT=on  SaturateOnIntegerOverflow=on  OutDataTypeStr=Inherit: Same as first input
  Sum3 : Sum  Inputs=-+  InputSameDT=on  SaturateOnIntegerOverflow=on  OutDataTypeStr=Inherit: Same as first input
  Sum7 : Sum  Inputs=+-  InputSameDT=on  SaturateOnIntegerOverflow=on  OutDataTypeStr=Inherit: Same as first input
  uBias : Constant  Value=u0
  out_u : Outport  VectorParamsAs1DForOutWhenUnconnected=off
  wires:
  Gain3/1 -> Sum/1
  Sum5/1 -> Integrator/1
  Gain9/1 -> Sum5/2
  Gain1/1 -> Sum5/1
  Sum3/1 -> Gain9/1
  Sum/1 -> Sum4/2
  Gain5/1 -> Sum2/1, Sum1/2
  Sum2/1 -> Gain3/1
  Gain7/1 -> Sum2/2, Sum1/1
  Sum1/1 -> Gain1/1
  in_y/1 -> Sum7/1, Gain5/1
  SP/1 -> Gain7/1
  Integrator/1 -> Sum/2
  uBias/1 -> Sum4/1
  in_yaw/1 -> Sum3/2
  Constant5/1 -> Saturation Dynamic/3
  Saturation Dynamic/1 -> Sum6/2  "q4corr"
  MIN/1 -> Sum7/2
  Gain2/1 -> Saturation Dynamic/2
  Sum7/1 -> Gain2/1
  Constant1/1 -> Saturation Dynamic/1
  Sum4/1 -> Sum3/1, Sum6/1
  Sum6/1 -> out_u/1

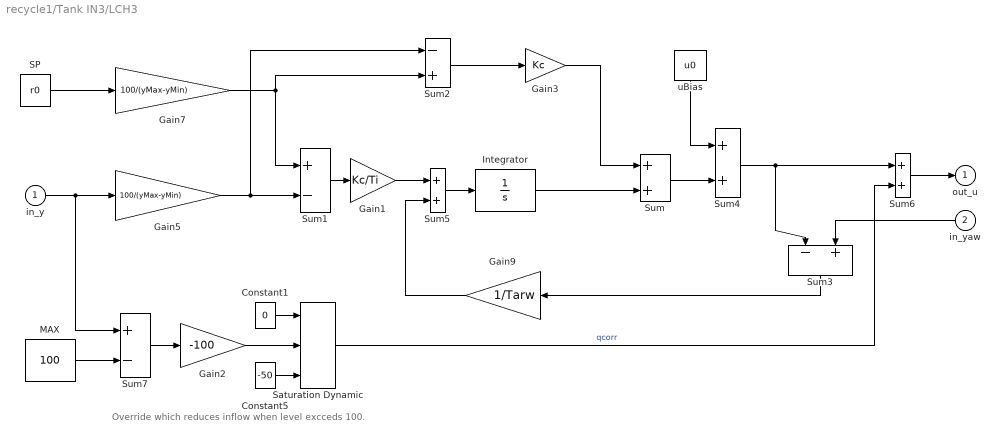
== system recycle1/Tank IN3/LCH3 ==
  note: Override which reduces inflow when level excceds 100.
  in_y : Inport
  in_yaw : Inport  Port=2
  Constant1 : Constant  Value=0
  Constant5 : Constant  Value=-50
  Gain1 : Gain  Gain=Kc/Ti  SaturateOnIntegerOverflow=on  OutDataTypeStr=Inherit: Same as input  ParamDataTypeStr=Inherit: Same as input
  Gain2 : Gain  Gain=-100  SaturateOnIntegerOverflow=on  OutDataTypeStr=Inherit: Same as input  ParamDataTypeStr=Inherit: Same as input
  Gain3 : Gain  Gain=Kc  SaturateOnIntegerOverflow=on  OutDataTypeStr=Inherit: Same as input  ParamDataTypeStr=Inherit: Same as input
  Gain5 : Gain  Gain=100/(yMax-yMin)  SaturateOnIntegerOverflow=on  OutDataTypeStr=Inherit: Same as input  ParamDataTypeStr=Inherit: Same as input
  Gain7 : Gain  Gain=100/(yMax-yMin)  SaturateOnIntegerOverflow=on  OutDataTypeStr=Inherit: Same as input  ParamDataTypeStr=Inherit: Same as input
  Gain9 : Gain  Gain=1/Tarw  SaturateOnIntegerOverflow=on  OutDataTypeStr=Inherit: Same as input  ParamDataTypeStr=Inherit: Same as input
  Integrator : Integrator
  MAX : Constant  Value=100
  SP : Constant  Value=r0
  Saturation Dynamic : simulink/Discontinuities/Saturation Dynamic  OutMin=[]  OutMax=[]  OutDataTypeStr=Inherit: Same as second input  OutDataType=fixdt(1, 16)  OutScaling=2^-10  DoSatur=off
  Sum{,4..6} (4 alike) : Sum  InputSameDT=on  SaturateOnIntegerOverflow=on  OutDataTypeStr=Inherit: Same as first input
  Sum1 : Sum  Inputs=+-  InputSameDT=on  SaturateOnIntegerOverflow=on  OutDataTypeStr=Inherit: Same as first input
  Sum2 : Sum  Inputs=-+  InputSameDT=on  SaturateOnIntegerOverflow=on  OutDataTypeStr=Inherit: Same as first input
  Sum3 : Sum  Inputs=-+  InputSameDT=on  SaturateOnIntegerOverflow=on  OutDataTypeStr=Inherit: Same as first input
  Sum7 : Sum  Inputs=+-  InputSameDT=on  SaturateOnIntegerOverflow=on  OutDataTypeStr=Inherit: Same as first input
  uBias : Constant  Value=u0
  out_u : Outport  VectorParamsAs1DForOutWhenUnconnected=off
  wires:
  Gain3/1 -> Sum/1
  Sum5/1 -> Integrator/1
  Gain9/1 -> Sum5/2
  Gain1/1 -> Sum5/1
  Sum3/1 -> Gain9/1
  Sum/1 -> Sum4/2
  Sum4/1 -> Sum6/1, Sum3/1
  Gain5/1 -> Sum2/1, Sum1/2
  Sum2/1 -> Gain3/1
  Gain7/1 -> Sum2/2, Sum1/1
  Sum1/1 -> Gain1/1
  in_y/1 -> Sum7/1, Gain5/1
  SP/1 -> Gain7/1
  Integrator/1 -> Sum/2
  uBias/1 -> Sum4/1
  in_yaw/1 -> Sum3/2
  Gain2/1 -> Saturation Dynamic/2
  Constant1/1 -> Saturation Dynamic/1
  Constant5/1 -> Saturation Dynamic/3
  Sum6/1 -> out_u/1
  Saturation Dynamic/1 -> Sum6/2  "qcorr"
  Sum7/1 -> Gain2/1
  MAX/1 -> Sum7/2

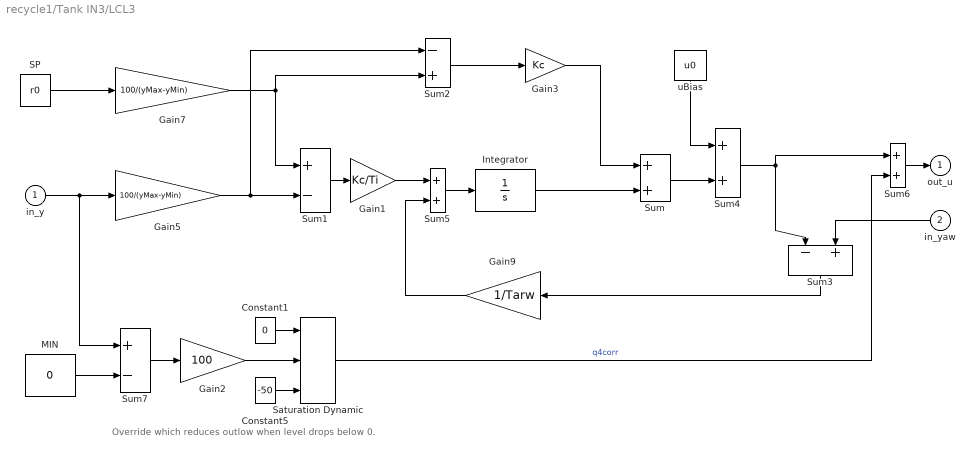
== system recycle1/Tank IN3/LCL3 ==
  note: Override which reduces outlow when level drops below 0.
  in_y : Inport
  in_yaw : Inport  Port=2
  Constant1 : Constant  Value=0
  Constant5 : Constant  Value=-50
  Gain1 : Gain  Gain=Kc/Ti  SaturateOnIntegerOverflow=on  OutDataTypeStr=Inherit: Same as input  ParamDataTypeStr=Inherit: Same as input
  Gain2 : Gain  Gain=100  SaturateOnIntegerOverflow=on  OutDataTypeStr=Inherit: Same as input  ParamDataTypeStr=Inherit: Same as input
  Gain3 : Gain  Gain=Kc  SaturateOnIntegerOverflow=on  OutDataTypeStr=Inherit: Same as input  ParamDataTypeStr=Inherit: Same as input
  Gain5 : Gain  Gain=100/(yMax-yMin)  SaturateOnIntegerOverflow=on  OutDataTypeStr=Inherit: Same as input  ParamDataTypeStr=Inherit: Same as input
  Gain7 : Gain  Gain=100/(yMax-yMin)  SaturateOnIntegerOverflow=on  OutDataTypeStr=Inherit: Same as input  ParamDataTypeStr=Inherit: Same as input
  Gain9 : Gain  Gain=1/Tarw  SaturateOnIntegerOverflow=on  OutDataTypeStr=Inherit: Same as input  ParamDataTypeStr=Inherit: Same as input
  Integrator : Integrator
  MIN : Constant  Value=0
  SP : Constant  Value=r0
  Saturation Dynamic : simulink/Discontinuities/Saturation Dynamic  OutMin=[]  OutMax=[]  OutDataTypeStr=Inherit: Same as second input  OutDataType=fixdt(1, 16)  OutScaling=2^-10  DoSatur=off
  Sum{,4..6} (4 alike) : Sum  InputSameDT=on  SaturateOnIntegerOverflow=on  OutDataTypeStr=Inherit: Same as first input
  Sum1 : Sum  Inputs=+-  InputSameDT=on  SaturateOnIntegerOverflow=on  OutDataTypeStr=Inherit: Same as first input
  Sum2 : Sum  Inputs=-+  InputSameDT=on  SaturateOnIntegerOverflow=on  OutDataTypeStr=Inherit: Same as first input
  Sum3 : Sum  Inputs=-+  InputSameDT=on  SaturateOnIntegerOverflow=on  OutDataTypeStr=Inherit: Same as first input
  Sum7 : Sum  Inputs=+-  InputSameDT=on  SaturateOnIntegerOverflow=on  OutDataTypeStr=Inherit: Same as first input
  uBias : Constant  Value=u0
  out_u : Outport  VectorParamsAs1DForOutWhenUnconnected=off
  wires:
  Gain3/1 -> Sum/1
  Sum5/1 -> Integrator/1
  Gain9/1 -> Sum5/2
  Gain1/1 -> Sum5/1
  Sum3/1 -> Gain9/1
  Sum/1 -> Sum4/2
  Gain5/1 -> Sum2/1, Sum1/2
  Sum2/1 -> Gain3/1
  Gain7/1 -> Sum2/2, Sum1/1
  Sum1/1 -> Gain1/1
  in_y/1 -> Sum7/1, Gain5/1
  SP/1 -> Gain7/1
  Integrator/1 -> Sum/2
  uBias/1 -> Sum4/1
  in_yaw/1 -> Sum3/2
  Constant5/1 -> Saturation Dynamic/3
  Saturation Dynamic/1 -> Sum6/2  "q4corr"
  MIN/1 -> Sum7/2
  Gain2/1 -> Saturation Dynamic/2
  Sum7/1 -> Gain2/1
  Constant1/1 -> Saturation Dynamic/1
  Sum4/1 -> Sum3/1, Sum6/1
  Sum6/1 -> out_u/1

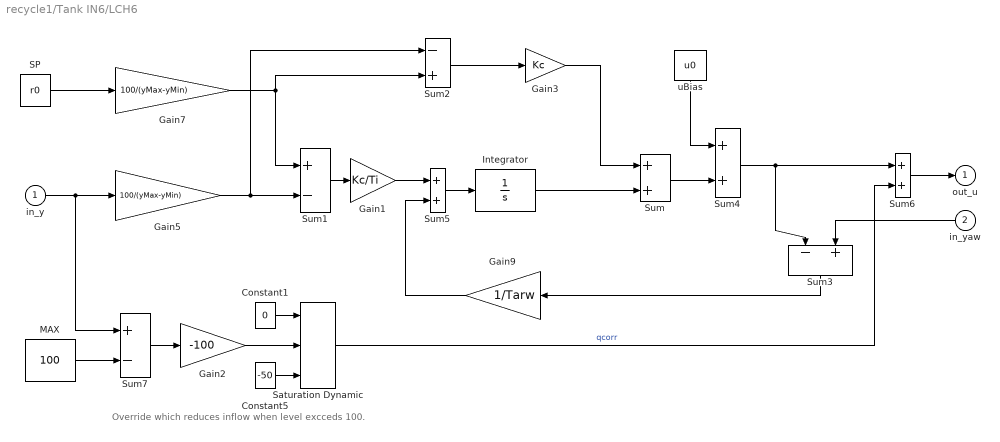
== system recycle1/Tank IN6/LCH6 ==
  note: Override which reduces inflow when level excceds 100.
  in_y : Inport
  in_yaw : Inport  Port=2
  Constant1 : Constant  Value=0
  Constant5 : Constant  Value=-50
  Gain1 : Gain  Gain=Kc/Ti  SaturateOnIntegerOverflow=on  OutDataTypeStr=Inherit: Same as input  ParamDataTypeStr=Inherit: Same as input
  Gain2 : Gain  Gain=-100  SaturateOnIntegerOverflow=on  OutDataTypeStr=Inherit: Same as input  ParamDataTypeStr=Inherit: Same as input
  Gain3 : Gain  Gain=Kc  SaturateOnIntegerOverflow=on  OutDataTypeStr=Inherit: Same as input  ParamDataTypeStr=Inherit: Same as input
  Gain5 : Gain  Gain=100/(yMax-yMin)  SaturateOnIntegerOverflow=on  OutDataTypeStr=Inherit: Same as input  ParamDataTypeStr=Inherit: Same as input
  Gain7 : Gain  Gain=100/(yMax-yMin)  SaturateOnIntegerOverflow=on  OutDataTypeStr=Inherit: Same as input  ParamDataTypeStr=Inherit: Same as input
  Gain9 : Gain  Gain=1/Tarw  SaturateOnIntegerOverflow=on  OutDataTypeStr=Inherit: Same as input  ParamDataTypeStr=Inherit: Same as input
  Integrator : Integrator
  MAX : Constant  Value=100
  SP : Constant  Value=r0
  Saturation Dynamic : simulink/Discontinuities/Saturation Dynamic  OutMin=[]  OutMax=[]  OutDataTypeStr=Inherit: Same as second input  OutDataType=fixdt(1, 16)  OutScaling=2^-10  DoSatur=off
  Sum{,4..6} (4 alike) : Sum  InputSameDT=on  SaturateOnIntegerOverflow=on  OutDataTypeStr=Inherit: Same as first input
  Sum1 : Sum  Inputs=+-  InputSameDT=on  SaturateOnIntegerOverflow=on  OutDataTypeStr=Inherit: Same as first input
  Sum2 : Sum  Inputs=-+  InputSameDT=on  SaturateOnIntegerOverflow=on  OutDataTypeStr=Inherit: Same as first input
  Sum3 : Sum  Inputs=-+  InputSameDT=on  SaturateOnIntegerOverflow=on  OutDataTypeStr=Inherit: Same as first input
  Sum7 : Sum  Inputs=+-  InputSameDT=on  SaturateOnIntegerOverflow=on  OutDataTypeStr=Inherit: Same as first input
  uBias : Constant  Value=u0
  out_u : Outport  VectorParamsAs1DForOutWhenUnconnected=off
  wires:
  Gain3/1 -> Sum/1
  Sum5/1 -> Integrator/1
  Gain9/1 -> Sum5/2
  Gain1/1 -> Sum5/1
  Sum3/1 -> Gain9/1
  Sum/1 -> Sum4/2
  Sum4/1 -> Sum6/1, Sum3/1
  Gain5/1 -> Sum2/1, Sum1/2
  Sum2/1 -> Gain3/1
  Gain7/1 -> Sum2/2, Sum1/1
  Sum1/1 -> Gain1/1
  in_y/1 -> Sum7/1, Gain5/1
  SP/1 -> Gain7/1
  Integrator/1 -> Sum/2
  uBias/1 -> Sum4/1
  in_yaw/1 -> Sum3/2
  Gain2/1 -> Saturation Dynamic/2
  Constant1/1 -> Saturation Dynamic/1
  Constant5/1 -> Saturation Dynamic/3
  Sum6/1 -> out_u/1
  Saturation Dynamic/1 -> Sum6/2  "qcorr"
  Sum7/1 -> Gain2/1
  MAX/1 -> Sum7/2

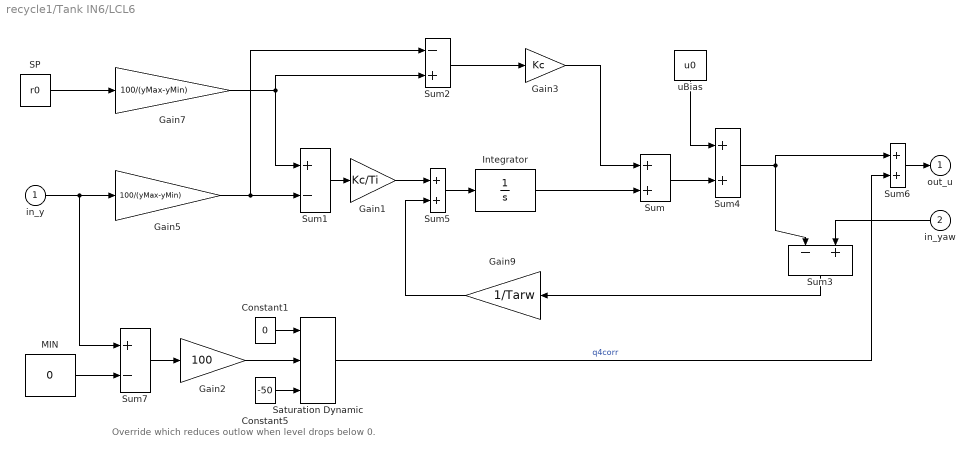
== system recycle1/Tank IN6/LCL6 ==
  note: Override which reduces outlow when level drops below 0.
  in_y : Inport
  in_yaw : Inport  Port=2
  Constant1 : Constant  Value=0
  Constant5 : Constant  Value=-50
  Gain1 : Gain  Gain=Kc/Ti  SaturateOnIntegerOverflow=on  OutDataTypeStr=Inherit: Same as input  ParamDataTypeStr=Inherit: Same as input
  Gain2 : Gain  Gain=100  SaturateOnIntegerOverflow=on  OutDataTypeStr=Inherit: Same as input  ParamDataTypeStr=Inherit: Same as input
  Gain3 : Gain  Gain=Kc  SaturateOnIntegerOverflow=on  OutDataTypeStr=Inherit: Same as input  ParamDataTypeStr=Inherit: Same as input
  Gain5 : Gain  Gain=100/(yMax-yMin)  SaturateOnIntegerOverflow=on  OutDataTypeStr=Inherit: Same as input  ParamDataTypeStr=Inherit: Same as input
  Gain7 : Gain  Gain=100/(yMax-yMin)  SaturateOnIntegerOverflow=on  OutDataTypeStr=Inherit: Same as input  ParamDataTypeStr=Inherit: Same as input
  Gain9 : Gain  Gain=1/Tarw  SaturateOnIntegerOverflow=on  OutDataTypeStr=Inherit: Same as input  ParamDataTypeStr=Inherit: Same as input
  Integrator : Integrator
  MIN : Constant  Value=0
  SP : Constant  Value=r0
  Saturation Dynamic : simulink/Discontinuities/Saturation Dynamic  OutMin=[]  OutMax=[]  OutDataTypeStr=Inherit: Same as second input  OutDataType=fixdt(1, 16)  OutScaling=2^-10  DoSatur=off
  Sum{,4..6} (4 alike) : Sum  InputSameDT=on  SaturateOnIntegerOverflow=on  OutDataTypeStr=Inherit: Same as first input
  Sum1 : Sum  Inputs=+-  InputSameDT=on  SaturateOnIntegerOverflow=on  OutDataTypeStr=Inherit: Same as first input
  Sum2 : Sum  Inputs=-+  InputSameDT=on  SaturateOnIntegerOverflow=on  OutDataTypeStr=Inherit: Same as first input
  Sum3 : Sum  Inputs=-+  InputSameDT=on  SaturateOnIntegerOverflow=on  OutDataTypeStr=Inherit: Same as first input
  Sum7 : Sum  Inputs=+-  InputSameDT=on  SaturateOnIntegerOverflow=on  OutDataTypeStr=Inherit: Same as first input
  uBias : Constant  Value=u0
  out_u : Outport  VectorParamsAs1DForOutWhenUnconnected=off
  wires:
  Gain3/1 -> Sum/1
  Sum5/1 -> Integrator/1
  Gain9/1 -> Sum5/2
  Gain1/1 -> Sum5/1
  Sum3/1 -> Gain9/1
  Sum/1 -> Sum4/2
  Gain5/1 -> Sum2/1, Sum1/2
  Sum2/1 -> Gain3/1
  Gain7/1 -> Sum2/2, Sum1/1
  Sum1/1 -> Gain1/1
  in_y/1 -> Sum7/1, Gain5/1
  SP/1 -> Gain7/1
  Integrator/1 -> Sum/2
  uBias/1 -> Sum4/1
  in_yaw/1 -> Sum3/2
  Constant5/1 -> Saturation Dynamic/3
  Saturation Dynamic/1 -> Sum6/2  "q4corr"
  MIN/1 -> Sum7/2
  Gain2/1 -> Saturation Dynamic/2
  Sum7/1 -> Gain2/1
  Constant1/1 -> Saturation Dynamic/1
  Sum4/1 -> Sum3/1, Sum6/1
  Sum6/1 -> out_u/1

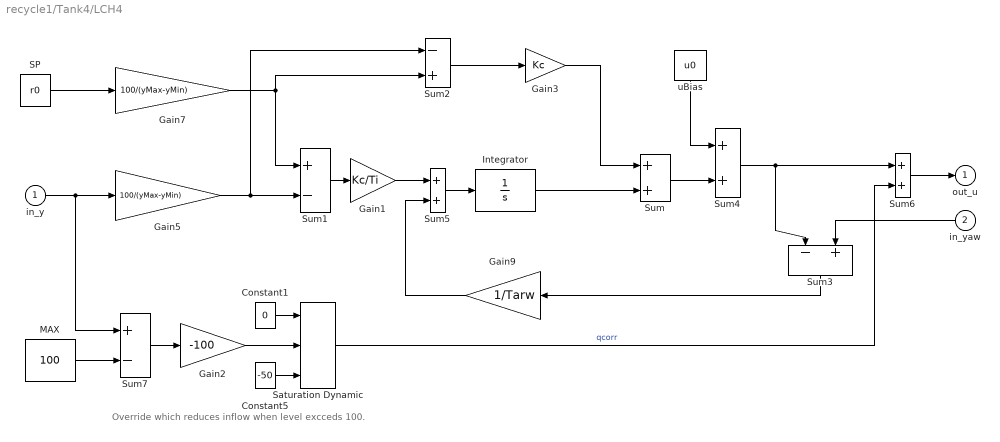
== system recycle1/Tank4/LCH4 ==
  note: Override which reduces inflow when level excceds 100.
  in_y : Inport
  in_yaw : Inport  Port=2
  Constant1 : Constant  Value=0
  Constant5 : Constant  Value=-50
  Gain1 : Gain  Gain=Kc/Ti  SaturateOnIntegerOverflow=on  OutDataTypeStr=Inherit: Same as input  ParamDataTypeStr=Inherit: Same as input
  Gain2 : Gain  Gain=-100  SaturateOnIntegerOverflow=on  OutDataTypeStr=Inherit: Same as input  ParamDataTypeStr=Inherit: Same as input
  Gain3 : Gain  Gain=Kc  SaturateOnIntegerOverflow=on  OutDataTypeStr=Inherit: Same as input  ParamDataTypeStr=Inherit: Same as input
  Gain5 : Gain  Gain=100/(yMax-yMin)  SaturateOnIntegerOverflow=on  OutDataTypeStr=Inherit: Same as input  ParamDataTypeStr=Inherit: Same as input
  Gain7 : Gain  Gain=100/(yMax-yMin)  SaturateOnIntegerOverflow=on  OutDataTypeStr=Inherit: Same as input  ParamDataTypeStr=Inherit: Same as input
  Gain9 : Gain  Gain=1/Tarw  SaturateOnIntegerOverflow=on  OutDataTypeStr=Inherit: Same as input  ParamDataTypeStr=Inherit: Same as input
  Integrator : Integrator
  MAX : Constant  Value=100
  SP : Constant  Value=r0
  Saturation Dynamic : simulink/Discontinuities/Saturation Dynamic  OutMin=[]  OutMax=[]  OutDataTypeStr=Inherit: Same as second input  OutDataType=fixdt(1, 16)  OutScaling=2^-10  DoSatur=off
  Sum{,4..6} (4 alike) : Sum  InputSameDT=on  SaturateOnIntegerOverflow=on  OutDataTypeStr=Inherit: Same as first input
  Sum1 : Sum  Inputs=+-  InputSameDT=on  SaturateOnIntegerOverflow=on  OutDataTypeStr=Inherit: Same as first input
  Sum2 : Sum  Inputs=-+  InputSameDT=on  SaturateOnIntegerOverflow=on  OutDataTypeStr=Inherit: Same as first input
  Sum3 : Sum  Inputs=-+  InputSameDT=on  SaturateOnIntegerOverflow=on  OutDataTypeStr=Inherit: Same as first input
  Sum7 : Sum  Inputs=+-  InputSameDT=on  SaturateOnIntegerOverflow=on  OutDataTypeStr=Inherit: Same as first input
  uBias : Constant  Value=u0
  out_u : Outport  VectorParamsAs1DForOutWhenUnconnected=off
  wires:
  Gain3/1 -> Sum/1
  Sum5/1 -> Integrator/1
  Gain9/1 -> Sum5/2
  Gain1/1 -> Sum5/1
  Sum3/1 -> Gain9/1
  Sum/1 -> Sum4/2
  Sum4/1 -> Sum6/1, Sum3/1
  Gain5/1 -> Sum2/1, Sum1/2
  Sum2/1 -> Gain3/1
  Gain7/1 -> Sum2/2, Sum1/1
  Sum1/1 -> Gain1/1
  in_y/1 -> Sum7/1, Gain5/1
  SP/1 -> Gain7/1
  Integrator/1 -> Sum/2
  uBias/1 -> Sum4/1
  in_yaw/1 -> Sum3/2
  Gain2/1 -> Saturation Dynamic/2
  Constant1/1 -> Saturation Dynamic/1
  Constant5/1 -> Saturation Dynamic/3
  Sum6/1 -> out_u/1
  Saturation Dynamic/1 -> Sum6/2  "qcorr"
  Sum7/1 -> Gain2/1
  MAX/1 -> Sum7/2
